simulink model "Boat_sim"  (Simulink 6.6)
settings: Solver=ode3  StartTime=0.0  StopTime=10000  FixedStep=T_step  RelTol=1e-3
values from neighbouring files (symbols this model uses):
  C_d_sea_surge = 340    [boat_constants.m]
  d_prop = .4572    (= 0.4572)    [boat_constants.m]
  e_0 = 0    [boat_constants.m]
  K_t = 0.5    [boat_constants.m]
  mass = 550    [boat_constants.m]
  n_0 = 0    [boat_constants.m]
  phi_0 = 0    [boat_constants.m]
  proportional_band = .5    (= 0.5)    [boat_constants.m]
  rho_w = 1.03e3    (= 1030)    [boat_constants.m]
  rudder_angle_dot_max = 10    [boat_constants.m]
  wheelbase = 3.27    [boat_constants.m]
undefined symbols (not defined in the file or in its folder): render_boat, rudder_angle_max
libraries: simulink x1
settings Model: Creator=Administrator  LastModifiedBy=Administrator  SimulationMode=accelerator

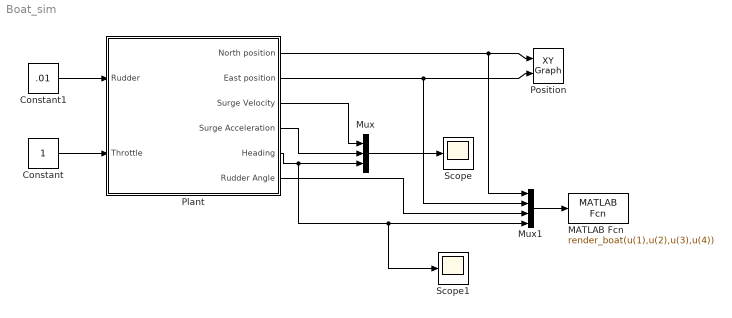
== system Boat_sim ==
  Constant : Constant
  Constant1 : Constant  Value=.01
  MATLAB Fcn : MATLABFcn  MATLABFcn=render_boat(u(1),u(2),u(3),u(4))  OutputDimensions=0  Output1D=off
  Mux : Mux  Inputs=3
  Mux1 : Mux
  Plant : Subsystem
  Position : simulink/Sinks/XY Graph  SystemSampleTime=-1  xmin=-1000  xmax=1000  ymin=-1000  ymax=1000  st=-1
  Scope : Scope
  Scope1 : Scope
  wires:
  Plant/1(North position) -> Mux1/1, Position/1
  Plant/2(East position) -> Mux1/2, Position/2
  Plant/3(Surge Velocity) -> Mux/1
  Plant/5(Heading) -> Mux1/4, Scope1/1, Mux/3
  Plant/4(Surge Acceleration) -> Mux/2
  Mux/1 -> Scope/1
  Mux1/1 -> MATLAB Fcn/1
  Plant/6(Rudder Angle) -> Mux1/3
  Constant/1 -> Plant/2(Throttle)
  Constant1/1 -> Plant/1(Rudder)

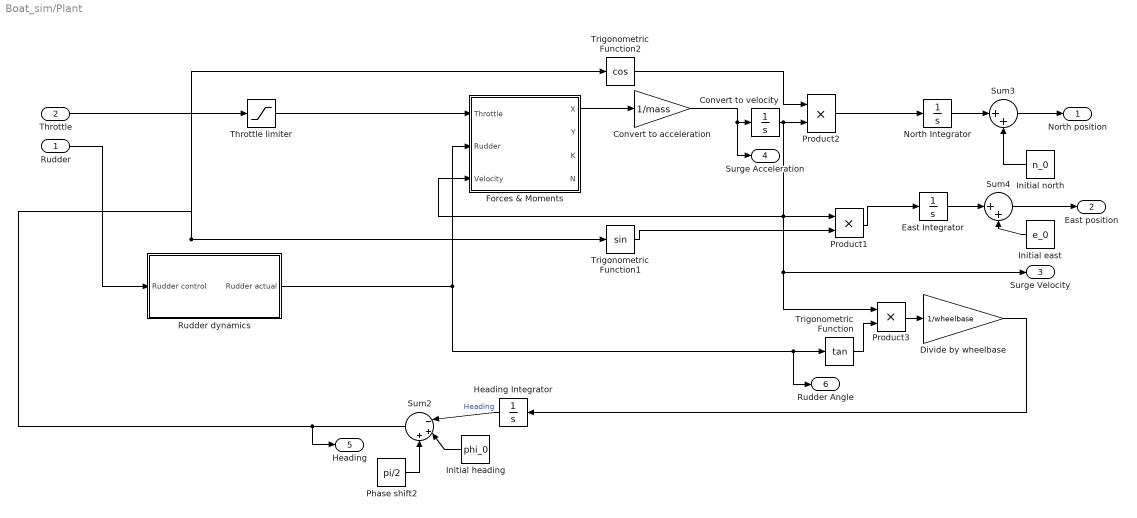
== system Boat_sim/Plant ==
  Rudder : Inport
  Throttle : Inport  Port=2
  Convert to acceleration : Gain  Gain=1/mass
  Convert to velocity : Integrator
  Divide by wheelbase : Gain  Gain=1/wheelbase
  East Integrator : Integrator
  Forces & Moments : Subsystem
  Heading Integrator : Integrator  Orientation=left
  Initial east : Constant  Orientation=left  Value=e_0
  Initial heading : Constant  Orientation=left  Value=phi_0
  Initial north : Constant  Orientation=left  Value=n_0
  North Integrator : Integrator
  Phase shift2 : Constant  Value=pi/2
  Product1 : Product  RndMeth=Zero
  Product2 : Product  RndMeth=Zero
  Product3 : Product  RndMeth=Zero
  Rudder dynamics : Subsystem
  Sum2 : Sum  Orientation=left  Inputs=|-++
  Sum3 : Sum  Inputs=|++
  Sum4 : Sum  Inputs=|++
  Throttle limiter : Saturate  UpperLimit=1  LowerLimit=0
  Trigonometric Function : Trigonometry  Operator=tan  OutputSignalType=real
  Trigonometric Function1 : Trigonometry  OutputSignalType=real
  Trigonometric Function2 : Trigonometry  Operator=cos  OutputSignalType=real
  North position : Outport
  East position : Outport  Port=2
  Surge Velocity : Outport  Port=3
  Surge Acceleration : Outport  Port=4
  Heading : Outport  Port=5
  Rudder Angle : Outport  Port=6
  wires:
  Trigonometric Function2/1 -> Product2/1
  Trigonometric Function/1 -> Product3/2
  Product3/1 -> Divide by wheelbase/1
  Product1/1 -> East Integrator/1
  Divide by wheelbase/1 -> Heading Integrator/1
  Convert to velocity/1 -> Product1/1, Product3/1, Forces & Moments/3(Velocity), Surge Velocity/1, Product2/2
  Convert to acceleration/1 -> Convert to velocity/1, Surge Acceleration/1
  Forces & Moments/1(X) -> Convert to acceleration/1
  Throttle/1 -> Throttle limiter/1
  Heading Integrator/1 -> Sum2/1  "Heading"
  Initial heading/1 -> Sum2/2
  Sum2/1 -> Heading/1, Trigonometric Function2/1, Trigonometric Function1/1
  Initial north/1 -> Sum3/2
  North Integrator/1 -> Sum3/1
  Sum3/1 -> North position/1
  East Integrator/1 -> Sum4/1
  Sum4/1 -> East position/1
  Initial east/1 -> Sum4/2
  Throttle limiter/1 -> Forces & Moments/1(Throttle)
  Phase shift2/1 -> Sum2/3
  Product2/1 -> North Integrator/1
  Trigonometric Function1/1 -> Product1/2
  Rudder/1 -> Rudder dynamics/1(Rudder control)
  Rudder dynamics/1(Rudder actual) -> Forces & Moments/2(Rudder), Trigonometric Function/1, Rudder Angle/1

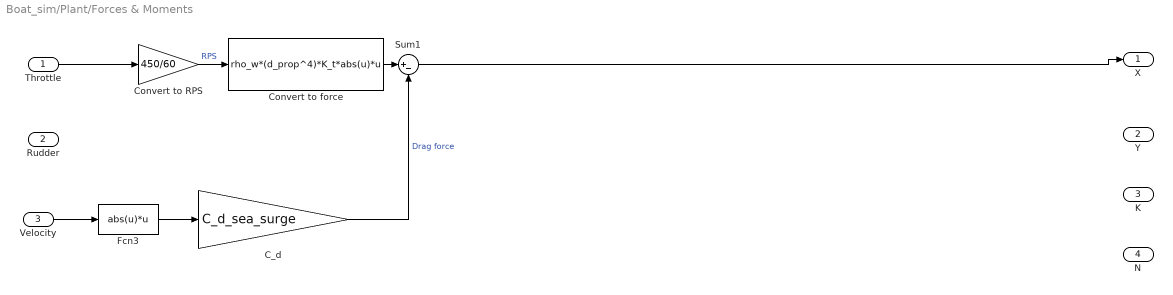
== system Boat_sim/Plant/Forces & Moments ==
  Throttle : Inport
  Rudder : Inport  Port=2
  Velocity : Inport  Port=3
  C_d : Gain  Gain=C_d_sea_surge
  Convert to RPS : Gain  Gain=450/60
  Convert to force : Fcn  Expr=rho_w*(d_prop^4)*K_t*abs(u)*u
  Fcn3 : Fcn  Expr=abs(u)*u
  Sum1 : Sum  Inputs=|+-
  X : Outport
  Y : Outport  Port=2
  K : Outport  Port=3
  N : Outport  Port=4
  wires:
  Convert to RPS/1 -> Convert to force/1  "RPS"
  Fcn3/1 -> C_d/1
  C_d/1 -> Sum1/2  "Drag force"
  Convert to force/1 -> Sum1/1
  Velocity/1 -> Fcn3/1
  Throttle/1 -> Convert to RPS/1
  Sum1/1 -> X/1

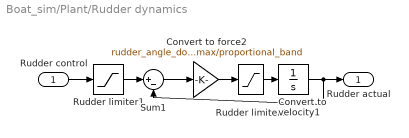
== system Boat_sim/Plant/Rudder dynamics ==
  Rudder control : Inport
  Convert to force2 : Gain  Gain=rudder_angle_dot_max/proportional_band
  Convert to velocity1 : Integrator  LimitOutput=on  UpperSaturationLimit=rudder_angle_max  LowerSaturationLimit=-rudder_angle_max
  Rudder limiter1 : Saturate  UpperLimit=rudder_angle_max  LowerLimit=-rudder_angle_max
  Rudder limiter2 : Saturate  UpperLimit=rudder_angle_dot_max  LowerLimit=-rudder_angle_dot_max
  Sum1 : Sum  Inputs=|+-
  Rudder actual : Outport
  wires:
  Convert to velocity1/1 -> Rudder actual/1, Sum1/2
  Sum1/1 -> Convert to force2/1
  Rudder limiter1/1 -> Sum1/1
  Rudder limiter2/1 -> Convert to velocity1/1
  Convert to force2/1 -> Rudder limiter2/1
  Rudder control/1 -> Rudder limiter1/1
